simulink model "Ball_Slope_Sim"  (Simulink 9.0)
settings: Solver=ode2  StartTime=0.0  StopTime=inf  FixedStep=0.005  RelTol=1e-3
InitFcn:
  | initialize
values from neighbouring files (symbols this model uses):
  c = 0    [initialize.m]
  C0 = [0 0 0]'    [initialize.m]
  g = 9.81    [initialize.m]
  k_lqr = lqr(A,B,QQ,RR)    [lqr_des.m]
  m = 1    [initialize.m]
  P0 = 1*eye(3)    [initialize.m]
  R = 1    [initialize.m]
  r = 0.1    [initialize.m]
  theta_eq = 0    [lqr_des.m]    (also in main.m = i*20)
  umax = 9*m    (= 9)    [initialize.m]
  umin = -9*m    (= -9)    [initialize.m]
  x0 = [theta0, dtheta0]'    [initialize.m]
libraries: simulink x4, sharedTrackingLibrary x1
settings Model: Creator=sihao  LastModifiedBy=samsun
settings DataIOCC: FinalStateName=myOperPoint  InitialState=myOperPoint  SaveCompleteFinalSimState=on  SaveFormat=Dataset
settings OptimizationCC: LifeSpan=auto
settings DebuggingCC: UnderspecifiedInitializationDetection=Simplified  MergeDetectMultiDrivingBlocksExec=error  SFUnexpectedBacktrackingDiag=error  SFNoUnconditionalDefaultTransitionDiag=error  SFExecutionAtInitializationDiag=warning
settings HardwareCC: ProdBitPerPointer=64  ProdBitPerSizeT=64  ProdBitPerPtrDiffT=64  ProdLargestAtomicFloat=Float  ProdIntDivRoundTo=Zero  ProdEndianess=LittleEndian  ProdWordSize=64  ProdHWDeviceType=Intel->x86-64 (Windows64)
settings ModelReferenceCC: PropagateSignalLabelsOutOfModel=on
settings CodeAppCC: StateflowObjectComments=off
settings GRTTargetCC: TargetLangStandard=C99 (ISO)
settings ConfigComp: CovMetricSettings=dwe  CovHtmlReporting=off  CovSaveCumulativeToWorkspaceVar=off  CovSaveSingleToWorkspaceVar=off  CovExternalEMLEnable=on

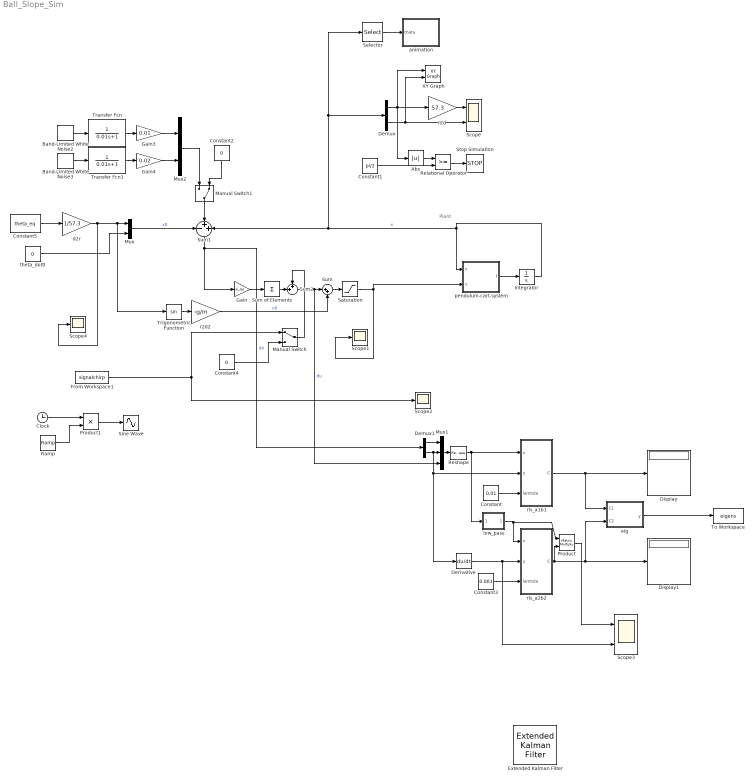
== system Ball_Slope_Sim ==
  note: Plant
  Abs : Abs
  Band-Limited White Noise2 : simulink/Sources/Band-Limited White Noise  Cov=[0.1]  Ts=0.1  seed=[23341]
  Band-Limited White Noise3 : simulink/Sources/Band-Limited White Noise  Cov=[0.1]  Ts=0.1  seed=[23341]
  Clock : Clock
  Constant : Constant  Value=0.01
  Constant1 : Constant  Value=pi/2
  Constant2 : Constant  Value=0
  Constant3 : Constant  Value=0.001
  Constant4 : Constant  Value=0
  Constant5 : Constant  Value=theta_eq
  Demux : Demux  Outputs=2
  Demux1 : Demux  Outputs=2
  Derivative : Derivative  CoefficientInTFapproximation=0.01
  Display : Display
  Display1 : Display
  Extended Kalman Filter : sharedTrackingLibrary/Extended Kalman Filter  StateTransitionFcn=myStateTransitionFcn  HasStateTransitionJacobianFcn=off  HasAdditiveProcessNoise=Additive  ProcessNoise=1  HasTimeVaryingProcessNoise=off  HasStateTransitionFcnExtraArgument=0  InitialState=0  InitialStateCovariance=1  MeasurementFcn1=myMeasurementFcn1  HasMeasurementJacobianFcn1=off  HasMeasurementEnablePort1=off  HasAdditiveMeasurementNoise1=Additive  MeasurementNoise1=1  HasTimeVaryingMeasurementNoise1=off  HasMeasurementFcnExtraArgument1=0  MeasurementFcn2=myMeasurementFcn2  HasMeasurementJacobianFcn2=off  HasMeasurementEnablePort2=off  HasAdditiveMeasurementNoise2=Additive  MeasurementNoise2=1  HasTimeVaryingMeasurementNoise2=off  HasMeasurementFcnExtraArgument2=0  MeasurementFcn3=myMeasurementFcn  HasMeasurementJacobianFcn3=off  HasMeasurementEnablePort3=off  HasAdditiveMeasurementNoise3=Additive  MeasurementNoise3=1  HasTimeVaryingMeasurementNoise3=off  HasMeasurementFcnExtraArgument3=0  MeasurementFcn4=myMeasurementFcn  HasMeasurementJacobianFcn4=off  HasMeasurementEnablePort4=off  HasAdditiveMeasurementNoise4=Additive  MeasurementNoise4=1  HasTimeVaryingMeasurementNoise4=off  HasMeasurementFcnExtraArgument4=0  MeasurementFcn5=myMeasurementFcn  HasMeasurementJacobianFcn5=off  HasMeasurementEnablePort5=off  HasAdditiveMeasurementNoise5=Additive  MeasurementNoise5=1  HasTimeVaryingMeasurementNoise5=off  HasMeasurementFcnExtraArgument5=0  EnableMultirate=off  StateTransitionFcnSampleTime=1  MeasurementFcn1SampleTime=1  MeasurementFcn2SampleTime=1  MeasurementFcn3SampleTime=1  MeasurementFcn4SampleTime=1  MeasurementFcn5SampleTime=1  UseCurrentEstimator=on  OutputStateCovariance=off  DataType=double  SampleTime=1  NumberOfMeasurements=2
      settings: SourceProductName=Control System Toolbox  SourceProductBaseCode=CT
  From Workspace1 : FromWorkspace  VariableName=signalchirp
  Gain : Gain  Gain=-k_lqr
  Gain3 : Gain  Gain=0.01
  Gain4 : Gain  Gain=0.02
  Integrator : Integrator  InitialCondition=x0
  Manual Switch : ManualSwitch
  Manual Switch1 : ManualSwitch  CurrentSetting=0
  Mux : Mux  Inputs=2
  Mux1 : Mux  Inputs=3
  Mux2 : Mux  Inputs=2
  Product : Product  Multiplication=Matrix(*)
  Product1 : Product
  Ramp : simulink/Sources/Ramp  slope=0.5  start=5  X0=0
  Relational Operator : RelationalOperator  OutDataTypeStr=boolean  RndMeth=Simplest
  Reshape : Reshape  OutputDimensionality=Row vector (2-D)
  Saturation : Saturate  UpperLimit=umax  LowerLimit=umin
  Scope : Scope  NumInputPorts=2
  Scope1 : Scope
  Scope2 : Scope
  Scope3 : Scope  NumInputPorts=2
  Scope4 : Scope
  Selector : Selector  InputPortWidth=2  IndexOptions=Index vector (dialog)  Indices=[1]  OutputSizes=1
  Sine Wave : Sin  TimeSource=Use external signal  SampleTime=0
  Stop Simulation : Stop
  Sum : Sum  Inputs=|++
  Sum of Elements : Sum  Inputs=+
  Sum1 : Sum  Inputs=-++
  Sum2 : Sum  Inputs=++|
  To Workspace : ToWorkspace  VariableName=eigens  SaveFormat=Timeseries  SampleTime=-1
  Transfer Fcn : TransferFcn  Denominator=[0.01 1]
  Transfer Fcn1 : TransferFcn  Denominator=[0.01 1]
  Trigonometric Function : Trigonometry
  XY Graph : simulink/Sinks/XY Graph  xmin=-5  xmax=5  ymin=-5  ymax=5  st=-1
  animation : MATLAB Function  TreatAsAtomicUnit=on
  d2r : Gain  Gain=1/57.3
  eig : MATLAB Function  TreatAsAtomicUnit=on
  low_pass : Subsystem
  pendulum-cart-system : MATLAB Function  TreatAsAtomicUnit=on
  r2d : Gain  Gain=57.3
  r2d2 : Gain  Gain=-g/m
  rls_a1b1 : Subsystem
  rls_a2b2 : Subsystem
  "theta_dot0 " : Constant  Value=0
  wires:
  Gain/1 -> Sum of Elements/1
  Demux/1 -> XY Graph/1, Abs/1, r2d/1
  Integrator/1 -> pendulum-cart-system/1(x), Sum1/3, Demux/1, Selector/1  "x"
  Selector/1 -> animation/1(theta)
  Constant1/1 -> Relational Operator/2
  Abs/1 -> Relational Operator/1
  Sum/1 -> Saturation/1
  r2d2/1 -> Sum/2  "u0"
  Demux/2 -> Scope/2, XY Graph/2
  Trigonometric Function/1 -> r2d2/1
  Mux/1 -> Sum1/1  "x0"
  Sum1/1 -> Demux1/1, Gain/1  "dx"
  Constant5/1 -> d2r/1
  "theta_dot0 "/1 -> Mux/2
  r2d/1 -> Scope/1
  Saturation/1 -> Scope1/1, pendulum-cart-system/2(u)
  Relational Operator/1 -> Stop Simulation/1
  Mux1/1 -> Reshape/1
  d2r/1 -> Scope4/1, Trigonometric Function/1, Mux/1
  Constant/1 -> rls_a1b1/3(lambda)
  rls_a1b1/1(C) -> eig/1(C1), Display/1
  From Workspace1/1 -> Manual Switch/1, Scope2/1
  Manual Switch/1 -> Sum2/1
  Constant4/1 -> Manual Switch/2
  Demux1/1 -> Mux1/1
  Demux1/2 -> rls_a1b1/2(y), Derivative/1, Mux1/2
  Reshape/1 -> rls_a1b1/1(x), low_pass/1(In1)
  Constant3/1 -> rls_a2b2/3(lambda)
  rls_a2b2/1(C) -> eig/2(C2), Display1/1, Product/2
  Sum2/1 -> Mux1/3, Sum/1  "du"
  Sum of Elements/1 -> Sum2/2
  Derivative/1 -> Scope3/2, rls_a2b2/2(y)
  pendulum-cart-system/1(f) -> Integrator/1
  Band-Limited White Noise3/1 -> Transfer Fcn1/1
  Band-Limited White Noise2/1 -> Transfer Fcn/1
  Gain3/1 -> Mux2/1
  Gain4/1 -> Mux2/2
  Mux2/1 -> Manual Switch1/1
  Transfer Fcn/1 -> Gain3/1
  Transfer Fcn1/1 -> Gain4/1
  Constant2/1 -> Manual Switch1/2
  Manual Switch1/1 -> Sum1/2
  Clock/1 -> Product1/1
  Ramp/1 -> Product1/2
  Product1/1 -> Sine Wave/1
  eig/1(y) -> To Workspace/1
  low_pass/1(Out1) -> Product/1, rls_a2b2/1(x)
  Product/1 -> Scope3/1

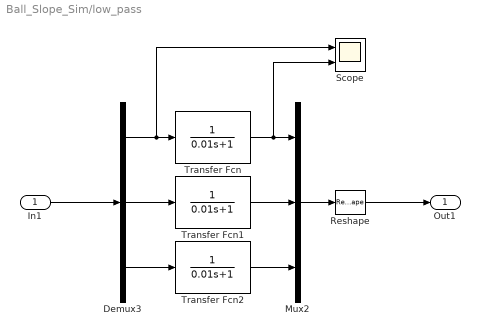
== system Ball_Slope_Sim/low_pass ==
  In1 : Inport
  Demux3 : Demux  Outputs=3
  Mux2 : Mux  Inputs=3
  Reshape : Reshape  OutputDimensionality=Row vector (2-D)
  Scope : Scope  NumInputPorts=2
  Transfer Fcn : TransferFcn  Denominator=[0.01 1]
  Transfer Fcn1 : TransferFcn  Denominator=[0.01 1]
  Transfer Fcn2 : TransferFcn  Denominator=[0.01 1]
  Out1 : Outport
  wires:
  Transfer Fcn2/1 -> Mux2/3
  Transfer Fcn1/1 -> Mux2/2
  Demux3/1 -> Scope/1, Transfer Fcn/1
  In1/1 -> Demux3/1
  Mux2/1 -> Reshape/1
  Demux3/2 -> Transfer Fcn1/1
  Demux3/3 -> Transfer Fcn2/1
  Transfer Fcn/1 -> Scope/2, Mux2/1
  Reshape/1 -> Out1/1

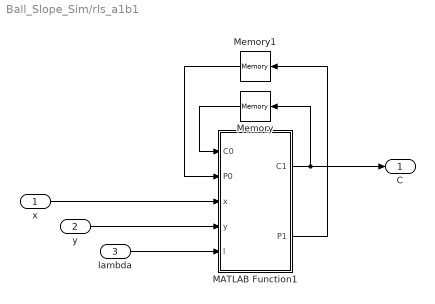
== system Ball_Slope_Sim/rls_a1b1 ==
  x : Inport
  y : Inport  Port=2
  lambda : Inport  Port=3
  MATLAB Function1 : MATLAB Function  TreatAsAtomicUnit=on  SystemSampleTime=0.1
  Memory : Memory  InitialCondition=C0
  Memory1 : Memory  InitialCondition=P0
  C : Outport
  wires:
  y/1 -> MATLAB Function1/4(y)
  x/1 -> MATLAB Function1/3(x)
  MATLAB Function1/2(P1) -> Memory1/1
  MATLAB Function1/1(C1) -> C/1, Memory/1
  Memory/1 -> MATLAB Function1/1(C0)
  Memory1/1 -> MATLAB Function1/2(P0)
  lambda/1 -> MATLAB Function1/5(l)

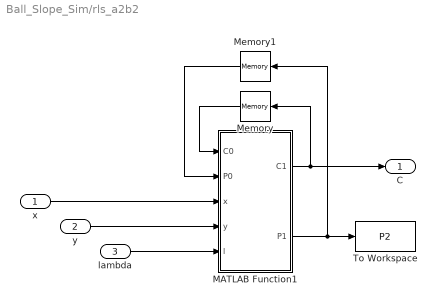
== system Ball_Slope_Sim/rls_a2b2 ==
  x : Inport
  y : Inport  Port=2
  lambda : Inport  Port=3
  MATLAB Function1 : MATLAB Function  TreatAsAtomicUnit=on  SystemSampleTime=0.1
  Memory : Memory  InitialCondition=C0
  Memory1 : Memory  InitialCondition=P0
  To Workspace : ToWorkspace  VariableName=P2  SaveFormat=Timeseries  SampleTime=-1
  C : Outport
  wires:
  lambda/1 -> MATLAB Function1/5(l)
  Memory1/1 -> MATLAB Function1/2(P0)
  Memory/1 -> MATLAB Function1/1(C0)
  MATLAB Function1/1(C1) -> Memory/1, C/1
  MATLAB Function1/2(P1) -> To Workspace/1, Memory1/1
  x/1 -> MATLAB Function1/3(x)
  y/1 -> MATLAB Function1/4(y)

== matlab function animation ==
  data: theta input double; R parameter double; r parameter double
function fcn(theta,R, r)


t = get(gca,'Children');

x = (R+r)*sin(theta);
y = (R+r)*cos(theta);
S = makehgtform('translate',[x y 0]);

set(t(2),'Matrix',S);

drawnow

end

== matlab function pendulum-cart-system ==
  data: x input double; u input double; f output double; m parameter double; R parameter double; c parameter double; g parameter double; sign parameter double
function f = fcn(x,u, m, R, c, g, sign)

% x(1): ball anglular position
% x(2): ball angular speed


f = zeros(2,1);

f(1) = x(2);
f(2) = sign*g*sin(x(1))/R  - c/m*x(2) + 1/(m*R)*u;


end

== matlab function rls_a2b2/MATLAB Function1 ==
  data: C0 input double; P0 input double; C1 output double; P1 output double; x input double; y input double; l input double
function [C1, P1] = fcn(C0, P0, x, y, l)
% RLS
% C0 : the last parameters;
% P0 : the last convariance matrix;
% x : the new measured regressor data;
% y : the new measurement;
% l : forgetting fector

K1 = P0*x'/(x*P0*x'+l);
C1 = C0+K1*(y-x*C0);
P1 = P0-K1*x*P0;

end

== matlab function rls_a1b1/MATLAB Function1 ==
  data: C0 input double; P0 input double; C1 output double; P1 output double; x input double; y input double; l input double
function [C1,P1] = fcn(C0,P0,x,y,l)
% RLS
% C0 : the last parameters;
% P0 : the last convariance matrix;
% x : the new measured regressor data;
% y : the new measurement;
% l : forgetting fector

K1 = P0*x'/(x*P0*x'+l);
C1 = C0+K1*(y-x*C0);
P1 = P0-K1*x*P0;

end

== matlab function eig ==
  data: C1 input double; y output double; C2 input double
function y = fcn(C1,C2)

A = [C1(1) C1(2); C2(1) C2(2)];

z = eig(A);

y = z;
end
